simulink model "arduino_buckboost"  (R2018b)
settings: Solver=ode3  StartTime=0.0  StopTime=Tmax*5  FixedStep=Tmax/10000  RelTol=1e-3
values from neighbouring files (symbols this model uses):
  a00c = sys(1).Ac(1,1)    [arduino_buckboost.m]    (also in arduino_buckboost_init.m)
  a00d = sys(1).Ad(1,1)    [arduino_buckboost.m]    (also in arduino_buckboost_init.m)
  a00o = sys(1).Ao(1,1)    [arduino_buckboost.m]    (also in arduino_buckboost_init.m)
  a01c = sys(1).Ac(1,2)    [arduino_buckboost.m]    (also in arduino_buckboost_init.m)
  a01d = sys(1).Ad(1,2)    [arduino_buckboost.m]    (also in arduino_buckboost_init.m)
  a01o = sys(1).Ao(1,2)    [arduino_buckboost.m]    (also in arduino_buckboost_init.m)
  a10c = sys(1).Ac(2,1)    [arduino_buckboost.m]    (also in arduino_buckboost_init.m)
  a10d = sys(1).Ad(2,1)    [arduino_buckboost.m]    (also in arduino_buckboost_init.m)
  a10o = sys(1).Ao(2,1)    [arduino_buckboost.m]    (also in arduino_buckboost_init.m)
  a11c = sys(1).Ac(2,2)    [arduino_buckboost.m]    (also in arduino_buckboost_init.m)
  a11d = sys(1).Ad(2,2)    [arduino_buckboost.m]    (also in arduino_buckboost_init.m)
  a11o = sys(1).Ao(2,2)    [arduino_buckboost.m]    (also in arduino_buckboost_init.m)
  b0c = sys(1).Bc(1)    [arduino_buckboost.m]    (also in arduino_buckboost_init.m)
  b0d = sys(1).Bd(1)    [arduino_buckboost.m]    (also in arduino_buckboost_init.m)
  b0o = sys(1).Bo(1)    [arduino_buckboost.m]    (also in arduino_buckboost_init.m)
  b1c = sys(1).Bc(2)    [arduino_buckboost.m]    (also in arduino_buckboost_init.m)
  b1d = sys(1).Bd(2)    [arduino_buckboost.m]    (also in arduino_buckboost_init.m)
  b1o = sys(1).Bo(2)    [arduino_buckboost.m]    (also in arduino_buckboost_init.m)
  i0 = single(i0)    [arduino_buckboost.m]    (also in arduino_buckboost_init.m)
  T = single(T)    [arduino_buckboost.m]    (also in arduino_buckboost_init.m)
  v0 = single(v0)    [arduino_buckboost.m]    (also in arduino_buckboost_init.m)
  Vref = single(Vref)    [arduino_buckboost.m]    (also in arduino_buckboost_init.m)
  Vs = single(Vs)    [arduino_buckboost.m]    (also in arduino_buckboost_init.m)
  Vs_noise = 0    [arduino_buckboost.m]    (also in arduino_buckboost_init.m)
  Vtol = single(Vtol)    [arduino_buckboost.m]    (also in arduino_buckboost_init.m)
libraries: arduinolib x3, realtime_examples_misc x1
settings Model: FPTRunName=Active  ExtModeTrigDuration=2  Creator=The MathWorks, Inc.  LastModifiedBy=taylo
settings SolverCC: AutoInsertRateTranBlk=on
settings DataIOCC: LimitDataPoints=on  SaveFormat=Array
settings OptimizationCC: DefaultParameterBehavior=Inlined  UseFloatMulNetSlope=on  DefaultUnderspecifiedDataType=single  InlineInvariantSignals=on  ExpressionDepthLimit=2147483647  EfficientFloat2IntCast=on  LifeSpan=Inf  MaxStackSize=64  OptimizeBlockOrder=speed
settings DebuggingCC: UnderspecifiedInitializationDetection=Classic  MergeDetectMultiDrivingBlocksExec=none  FcnCallInpInsideContextMsg=warning  AllowSymbolicDim=off  StateNameClashWarn=warning  LibraryContextMissingDiagnostic=none  SFUnexpectedBacktrackingDiag=warning  SFNoUnconditionalDefaultTransitionDiag=warning  SFExecutionAtInitializationDiag=none
settings HardwareCC: ProdBitPerInt=16  ProdBitPerPointer=16  ProdBitPerSizeT=16  ProdBitPerPtrDiffT=16  ProdLargestAtomicFloat=None  ProdWordSize=8  ProdLongLongMode=on  ProdHWDeviceType=Atmel->AVR
settings ModelReferenceCC: PropagateSignalLabelsOutOfModel=off  SupportModelReferenceSimTargetCustomCode=on
settings SFSimCC: SimUseLocalCustomCode=off  MATLABDynamicMemAlloc=off
settings RTWCC: SystemTargetFile=ert.tlc  HardwareBoard=Arduino Uno  PackageGeneratedCodeAndArtifacts=on  PackageName=all_out.zip  TemplateMakefile=ert_default_tmf  GenerateReport=on  RetainRTWFile=on  RTWUseLocalCustomCode=off  Toolchain=Arduino AVR  BuildConfiguration=Specify  LaunchReport=on
settings CodeAppCC: ForceParamTrailComments=on  OperatorAnnotations=on  StateflowObjectComments=on  MATLABSourceComments=on
settings ERTTargetCC: MultiwordLength=2048  CombineSignalStateStructs=on  ERTCustomFileBanners=off  SupportContinuousTime=on  SupportNonInlinedSFcns=on  RemoveResetFunc=off  SupportVariableSizeSignals=on  ModelStepFunctionPrototypeControlCompliant=off
settings ConfigComp: CovMetricSettings=dw  CovHtmlReporting=on  CovSaveCumulativeToWorkspaceVar=on  CovSaveSingleToWorkspaceVar=on  CovExternalEMLEnable=off  CovSFcnEnable=off

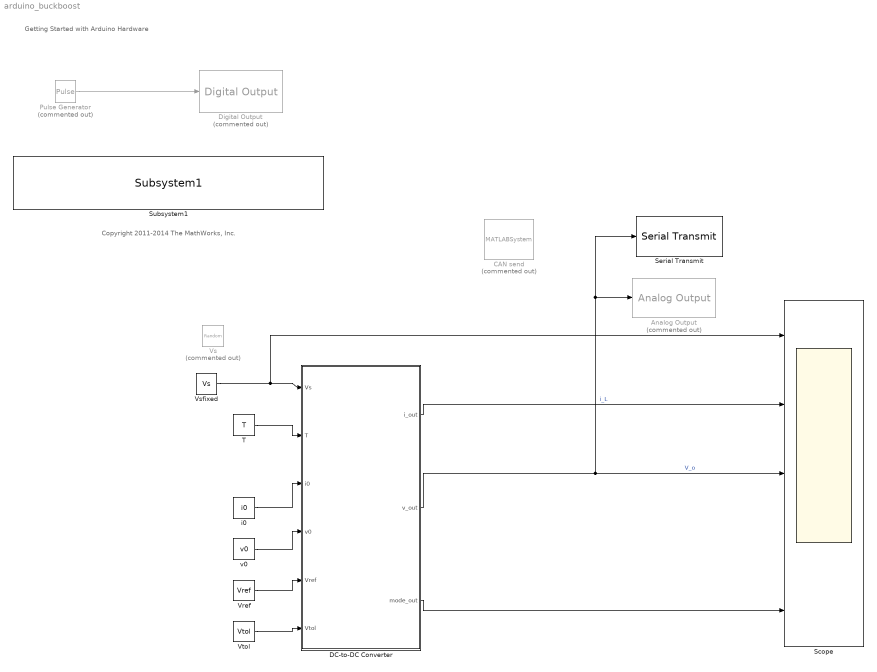
== system arduino_buckboost ==
  note: Getting Started with Arduino Hardware
  note: Copyright 2011-2014 The MathWorks, Inc.
  Analog Output : arduinolib/Analog Output  Commented=on  DACpin=DAC0  blockPlatform=arduino
      settings: SourceProductName=Simulink Support Package for Arduino Hardware  SourceProductBaseCode=ARDUINO
  CAN send : MATLABSystem  Commented=on  System=ArduinoCan
      mask Type: ArduinoCan
      mask Display:
      | disp('Sink');
      | port_label('input',1,'u');
  DC-to-DC Converter : Stateflow chart  TreatAsAtomicUnit=on
  Digital Output : arduinolib/Digital Output  Commented=on  pinNumber=9  blockPlatform=arduino
  Pulse Generator : DiscretePulseGenerator  Commented=on  Period=10  PulseWidth=5  SampleTime=0.1
  Scope : Scope  NumInputPorts=5
  Serial Transmit : arduinolib/Serial Transmit  portNumber=0  sendmode=println  label=vc  sendformat=Decimal  floatprecision=4  blockPlatform=arduino
      settings: SourceProductName=Simulink Support Package for Arduino Hardware
  Subsystem1 : realtime_examples_misc/Subsystem1  SystemSampleTime=-1
  T : Constant  Value=T
  Vref : Constant  Value=Vref
  Vs : RandomNumber  Commented=on  Mean=Vs  Variance=Vs_noise  SampleTime=0.0001
  Vsfixed : Constant  Value=Vs
  Vtol : Constant  Value=Vtol
  i0 : Constant  Value=i0
  v0 : Constant  Value=v0
  wires:
  Pulse Generator/1 -> Digital Output/1
  DC-to-DC Converter/1(i_out) -> Scope/2  "i_L"
  i0/1 -> DC-to-DC Converter/3(i0)
  Vtol/1 -> DC-to-DC Converter/6(Vtol)
  Vref/1 -> DC-to-DC Converter/5(Vref)
  DC-to-DC Converter/3(mode_out) -> Scope/5
  T/1 -> DC-to-DC Converter/2(T)
  v0/1 -> DC-to-DC Converter/4(v0)
  DC-to-DC Converter/2(v_out) -> Scope/3, Serial Transmit/1, Analog Output/1  "V_o"
  Vsfixed/1 -> Scope/1, DC-to-DC Converter/1(Vs)

== stateflow chart arduino_buckboost/DC-to-DC Converter ==
  settings: updateMethod=CONTINUOUS
  state Discontinuous
    du:
    i_dot = a00d*i+a01d*v+b0d*Vs;
    v_dot = a10d*i+a11d*v+b1d*Vs;
    t_dot = 1;
    i_out =i;
    v_out = v;
    mode_out=3;
  state Charging
    du:
    i_dot = a00c*i+a01c*v+b0c*Vs;
    v_dot = a10c*i+a11c*v+b1c*Vs;
    t_dot = 1;
    i_out = i;
    v_out = v;
    mode_out=2;
  state Discharging
    du:
    i_dot = a00o*i+a01o*v+b0o*Vs;
    v_dot = a10o*i+a11o*v+b1o*Vs;
    t_dot = 1;
    i_out = i;
    v_out = v;
    mode_out=1;
  Discharging -> Discontinuous [order 1] : [i <= 0]
  Discontinuous -> Charging : [v <= Vref-Vtol]
  Charging -> Discharging : [v >= Vref+Vtol]
  Discharging -> Charging [order 2] : [v <= Vref-Vtol]
  (default) -> Charging : {i = i0;
      | v = v0;}
  data: t local fixdt(0,16,15); i_out output single; v_out output single; i local fixdt(1,16,1); a00o local single =a00o; Vs input single =120; T input single; a01o local single =a01o; a10o local single =a10o; a11o local single =a11o; a00c local single =a00c; a01c local single =a01c; a10c local single =a10c; a11c local single =a11c; b0o local single =b0o; b1o local single =b1o; b0c local single =b0c; b1c local single =b1c; v local fixdt(1,16,2); i0 input single; v0 input single; a01d local single =a01d; a10d local single =a10d; a11d local single =a11d; a00d local single =a00d; b0d local single =b0d; b1d local single =b1d; Vref input single =120; mode_out output single; Vtol input single =120
  data t settings: updateMethod=SF_CONTINUOUS_TIME_DATA
  data i settings: updateMethod=SF_CONTINUOUS_TIME_DATA
  data v settings: updateMethod=SF_CONTINUOUS_TIME_DATA
  data Vtol settings: description=Voltage tolerance (e.g., Vref / 100 is +/- 1% voltage ripple)
